simulink model "uas_demo"  (R2021a)
settings: Solver=FixedStepAuto  StartTime=0.0  StopTime=Inf  FixedStep=sample_time  RelTol=1e-3
model workspace: external: MAT-File (data not in the file)
values from neighbouring files (symbols this model uses):
  arm_length = 0.225    [Quadcopter_setup_parameters.m]    (also in recording.mat = 0.17; uas_parameters.m = 0.17; uas_parameters.mat = 0.17)
  drag_coefficient = 0.47    [Quadcopter_setup_parameters.m]    (also in recording.mat; uas_parameters.m; uas_parameters.mat)
  g = 9.81    [Quadcopter_setup_parameters.m]    (also in recording.mat = 9.80665; uas_parameters.m = 9.80665; uas_parameters.mat = 9.80665)
  inertia_xx = 5*10^(-3)    (= 0.005)    [Quadcopter_setup_parameters.m]    (also in recording.mat = 0.007; uas_parameters.m = 0.007; uas_parameters.mat = 0.007)
  inertia_yy = 5*10^(-3)    (= 0.005)    [Quadcopter_setup_parameters.m]    (also in recording.mat = 0.007; uas_parameters.m = 0.007; uas_parameters.mat = 0.007)
  inertia_zz = 8.9*10^(-3)    (= 0.0089)    [Quadcopter_setup_parameters.m]    (also in recording.mat = 0.012; uas_parameters.m = 0.012; uas_parameters.mat = 0.012)
  m = 0.55    [Quadcopter_setup_parameters.m]
  mass_drone = 0.55    [Quadcopter_setup_parameters.m]    (also in recording.mat = 0.68; uas_parameters.m = 0.68; uas_parameters.mat = 0.68)
  mass_total = mass_drone + mass_rod + mass_tip    (= 0.55)    [Quadcopter_setup_parameters.m]    (also in recording.mat = 0.68; uas_parameters.m = 0.68; uas_parameters.mat = 0.68)
  max_rot_velocity = 838    [Quadcopter_setup_parameters.m]    (also in recording.mat; uas_parameters.m; uas_parameters.mat)
  mix_matrix = inv(motor_constant * allocation_matrix)    [Quadcopter_setup_parameters.m]    (also in recording.mat = [29244.6230836 29244.6230836 29244.6230836 29244.6230836 -5.; uas_parameters.m; uas_parameters.mat = [29244.6230836 29244.6230836 29244.6230836 29244.6230836 -5.)
  moment_constant = 0.1    [Quadcopter_setup_parameters.m]    (also in recording.mat = 0.016; uas_parameters.m = 0.016; uas_parameters.mat = 0.016)
  motor_constant = 0.01    [Quadcopter_setup_parameters.m]    (also in recording.mat = 8.54858e-06; uas_parameters.m = 8.54858e-06; uas_parameters.mat = 8.54858e-06)
  p1 = 13.0908027334    [recording.mat]    (also in uas_parameters.mat = 12.1300541038; uas_thrust.mat = 12.1300541038; uas_thrust_constants.mat = 11.8019985126; uas_thrust_identification.m = result.p1)
  p2 = 0.438838137767    [recording.mat]    (also in uas_parameters.mat = 1.4832987942; uas_thrust.mat = 1.4832987942; uas_thrust_constants.mat = 1.1585190761; uas_thrust_identification.m = result.p2)
  poly_traj = PolyTrajGen(knots, order, optimization_target, dim, max_continuity)    [uas_minimum_snap.m]    (also in uas_trajectory.m = uas_minimum_snap(knots, order, waypoints, velocities, corrid)
  publish_rate = 1 * sample_time    (= 0.001)    [Quadcopter_setup_parameters.m]    (also in recording.mat = 0.04; uas_parameters.m = 0.04; uas_parameters.mat = 0.04)
  reference_area = pi * 75e-3^2    (= 0.0176714586764)    [Quadcopter_setup_parameters.m]    (also in recording.mat; uas_parameters.m; uas_parameters.mat)
  rotor_offset_top = 0.01    [Quadcopter_setup_parameters.m]    (also in recording.mat; uas_parameters.m; uas_parameters.mat)
  sample_time = 1e-3    (= 0.001)    [Quadcopter_setup_parameters.m]    (also in recording.mat = 0.04; uas_parameters.m = 0.04; uas_parameters.mat = 0.04)
  X = 3    [Quadcopter_setup_parameters.m]
  x0 = 36    [Quadcopter_setup_parameters.m]    (also in recording.mat; uas_parameters.m; uas_parameters.mat)
  Y = 2    [Quadcopter_setup_parameters.m]
  y0 = 80    [Quadcopter_setup_parameters.m]    (also in recording.mat; uas_parameters.m; uas_parameters.mat)
  Z = 1    [Quadcopter_setup_parameters.m]
  z0 = 1    [Quadcopter_setup_parameters.m]    (also in recording.mat = 0.3; uas_parameters.m; uas_parameters.mat)
undefined symbols (not defined in the file or in its folder): Angular, Linear, Pose, Position, Twist
libraries: nesl_utility x32, sm_lib x25, robotlib x13, simulink_extras x6, vrlib x1, sim3dlib x1, uavsim3dlib x1
(part 3 of 3)

== matlab function uas_demo/quadcopter/real drone/get R33 ==
  data: q input; R33 output
function R33 = get_R33(q)

if norm(q, 2) > 0.5
    R = quat2rotm(q);
    R33 = R(3, 3);
else
    R33 = 1;
end

== matlab function uas_demo/quadcopter/simulated drone/Subsystem/MATLAB Function1 ==
  data: roll input size=1; pitch input size=1; yaw input size=1; er output size=[3 1]; R input size=[3 3]
function er = lee(roll, pitch, yaw, R)

Rd = eul2rotm([yaw pitch roll], 'ZYX');

P = 1/2 * (Rd.' * R - R.' * Rd) ;

er = [P(3,2) ; P(1,3) ; P(2,1)] ;

== matlab function uas_demo/quadcopter/real drone/quat 2 euler (ROS) ==
  data: q input size=[1 4]; roll_rad output; pitch_rad output; yaw_rad output
function [roll_rad, pitch_rad, yaw_rad] = euler_ros(q)

attitude = quat2eul(q, 'ZYX');

roll_rad = attitude(3);
pitch_rad = attitude(2);
yaw_rad = attitude(1);

== matlab function uas_demo/quadcopter/simulated drone/q2r ==
  data: q input; R output
function R = q2r(q)

if norm(q, 2) > 0.5
    R = quat2rotm(q);
else
    R = eye(3);
end

== matlab function uas_demo/trajectory generator/desired yaw ==
  data: v input; setpoint_yaw output; a input; setpoint_yaw_rate output
function [setpoint_yaw, setpoint_yaw_rate] = forward_yaw(v, a)

setpoint_yaw = atan2(v(2), v(1));
setpoint_yaw_rate = (-v(2)*a(1) + v(1)*a(2))/(v(1)^2 + v(2)^2);

== matlab function uas_demo/quadcopter/simulated drone/quat 2 euler (UE) ==
  data: q input size=[1 4]; attitude output
function attitude = euler_ue(q)

attitude = quat2eul(q, 'ZYX');

attitude = [attitude(1) attitude(2) attitude(3)];

== matlab function uas_demo/quadcopter/position controller/compute_roll_pitch ==
  data: F_d input; roll output; yaw_d input; pitch output
function [roll, pitch] = compute_roll_pitch(F_d, yaw_d)

yaw_dt = yaw_d + pi/2;
uyt = [cos(yaw_dt); sin(yaw_dt); 0];
uz = F_d/norm(F_d);
ux = cross(uyt, uz);
uy = cross(uz, ux);

attitude = rotm2eul([ux uy uz], 'ZYX');

roll = attitude(3);
pitch = attitude(2);
